simulink model "BiegeMaschineAllein"  (R2015b)
settings: Solver=ode45  StartTime=0.0  StopTime=10  RelTol=1e-3
libraries: simulink x8
settings Model: Creator=taprudho  LastModifiedBy=taprudho
settings DataIOCC: SaveFormat=Array  SignalLoggingSaveFormat=ModelDataLogs
settings OptimizationCC: ExpressionDepthLimit=2147483647
settings DebuggingCC: UnderspecifiedInitializationDetection=Classic  MergeDetectMultiDrivingBlocksExec=none  SolverPrmCheckMsg=warning  FcnCallInpInsideContextMsg=UseLocalSettings  StateNameClashWarn=warning  StrictBusMsg=Warning
settings HardwareCC: ProdBitPerPointer=32  ProdLargestAtomicFloat=None  ProdIntDivRoundTo=Undefined  ProdEndianess=Unspecified  ProdWordSize=32  ProdHWDeviceType=32-bit Generic
settings SFSimCC: SimParseCustomCode=off
settings GRTTargetCC: GeneratePreprocessorConditionals=Disable all  CombineOutputUpdateFcns=off  GRTInterface=on
settings ConfigComp: CovModelRefEnable=Off  CovSFcnEnable=off

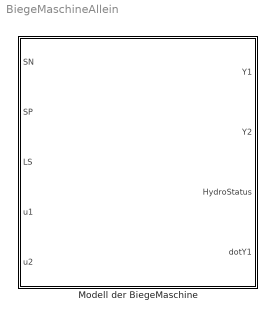
== system BiegeMaschineAllein ==
  Modell der BiegeMaschine : Subsystem

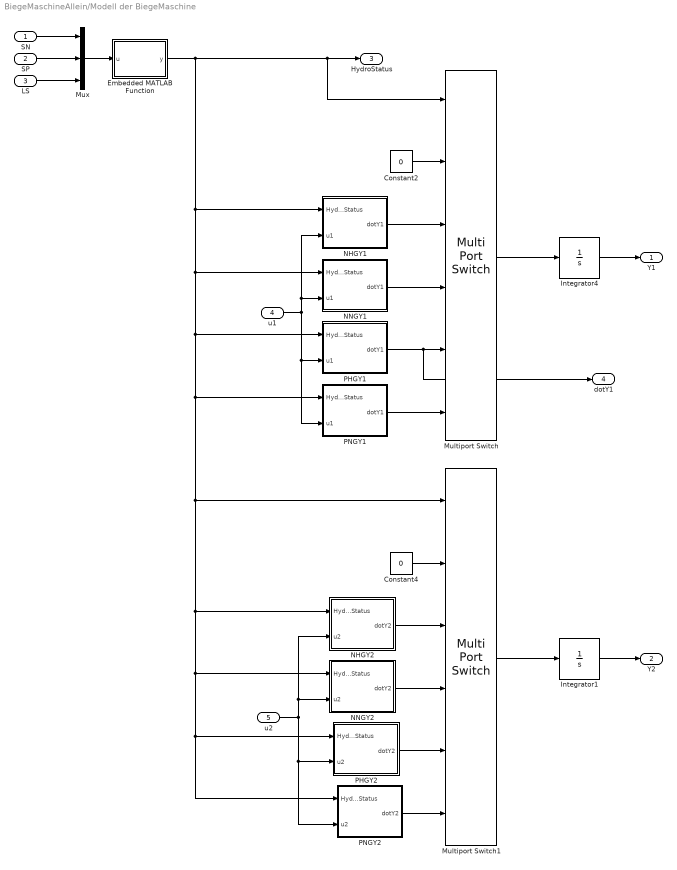
== system BiegeMaschineAllein/Modell der BiegeMaschine ==
  SN : Inport
  SP : Inport  Port=2
  LS : Inport  Port=3
  u1 : Inport  Port=4
  u2 : Inport  Port=5
  Constant2 : Constant  Value=0
  Constant4 : Constant  Value=0
  Embedded MATLAB Function : MATLAB Function  TreatAsAtomicUnit=on
  Integrator1 : Integrator
  Integrator4 : Integrator
  Multiport Switch : MultiPortSwitch  Inputs=5
  Multiport Switch1 : MultiPortSwitch  Inputs=5
  Mux : Mux  Inputs=3
  NHGY1 : Subsystem
  NHGY2 : Subsystem
  NNGY1 : Subsystem
  NNGY2 : Subsystem
  PHGY1 : Subsystem
  PHGY2 : Subsystem
  PNGY1 : Subsystem
  PNGY2 : Subsystem
  Y1 : Outport
  Y2 : Outport  Port=2
  HydroStatus : Outport  Port=3
  dotY1 : Outport  Port=4
  wires:
  SN/1 -> Mux/1
  SP/1 -> Mux/2
  LS/1 -> Mux/3
  Mux/1 -> Embedded MATLAB Function/1(u)
  Embedded MATLAB Function/1(y) -> Multiport Switch/1, HydroStatus/1, NHGY1/1(HydroStatus), NNGY1/1(HydroStatus), PHGY1/1(HydroStatus), Multiport Switch1/1, NHGY2/1(HydroStatus), NNGY2/1(HydroStatus), PHGY2/1(HydroStatus), PNGY2/1(HydroStatus), PNGY1/1(HydroStatus)
  NHGY1/1(dotY1) -> Multiport Switch/3
  NNGY1/1(dotY1) -> Multiport Switch/4
  PHGY1/1(dotY1) -> Multiport Switch/5, dotY1/1
  PNGY1/1(dotY1) -> Multiport Switch/6
  Constant2/1 -> Multiport Switch/2
  Multiport Switch/1 -> Integrator4/1
  Integrator4/1 -> Y1/1
  Constant4/1 -> Multiport Switch1/2
  NHGY2/1(dotY2) -> Multiport Switch1/3
  NNGY2/1(dotY2) -> Multiport Switch1/4
  PHGY2/1(dotY2) -> Multiport Switch1/5
  u2/1 -> NHGY2/2(u2), NNGY2/2(u2), PHGY2/2(u2), PNGY2/2(u2)
  Multiport Switch1/1 -> Integrator1/1
  Integrator1/1 -> Y2/1
  PNGY2/1(dotY2) -> Multiport Switch1/6
  u1/1 -> NHGY1/2(u1), NNGY1/2(u1), PHGY1/2(u1), PNGY1/2(u1)

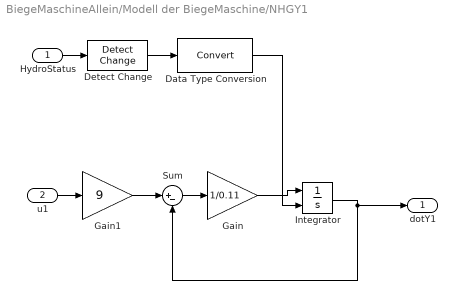
== system BiegeMaschineAllein/Modell der BiegeMaschine/NHGY1 ==
  HydroStatus : Inport
  u1 : Inport  Port=2
  Data Type Conversion : DataTypeConversion
  Detect Change : simulink/Logic and Bit Operations/Detect Change  vinit=0  InputProcessing=Inherited  OutDataTypeStr=uint8
  Gain : Gain  Gain=1/0.11
  Gain1 : Gain  Gain=9
  Integrator : Integrator  ExternalReset=either
  Sum : Sum  Inputs=|+-
  dotY1 : Outport
  wires:
  Gain/1 -> Integrator/1
  Sum/1 -> Gain/1
  Gain1/1 -> Sum/1
  Integrator/1 -> Sum/2, dotY1/1
  HydroStatus/1 -> Detect Change/1
  u1/1 -> Gain1/1
  Detect Change/1 -> Data Type Conversion/1
  Data Type Conversion/1 -> Integrator/2

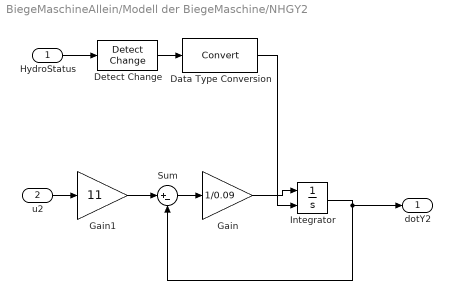
== system BiegeMaschineAllein/Modell der BiegeMaschine/NHGY2 ==
  HydroStatus : Inport
  u2 : Inport  Port=2
  Data Type Conversion : DataTypeConversion
  Detect Change : simulink/Logic and Bit Operations/Detect Change  SystemSampleTime=-1  vinit=0
  Gain : Gain  Gain=1/0.09
  Gain1 : Gain  Gain=11
  Integrator : Integrator  ExternalReset=either
  Sum : Sum  Inputs=|+-
  dotY2 : Outport
  wires:
  Gain/1 -> Integrator/1
  Sum/1 -> Gain/1
  Gain1/1 -> Sum/1
  Integrator/1 -> Sum/2, dotY2/1
  HydroStatus/1 -> Detect Change/1
  u2/1 -> Gain1/1
  Detect Change/1 -> Data Type Conversion/1
  Data Type Conversion/1 -> Integrator/2

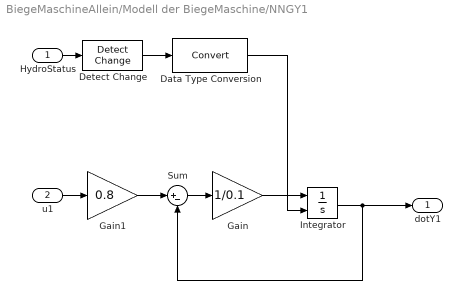
== system BiegeMaschineAllein/Modell der BiegeMaschine/NNGY1 ==
  HydroStatus : Inport
  u1 : Inport  Port=2
  Data Type Conversion : DataTypeConversion
  Detect Change : simulink/Logic and Bit Operations/Detect Change  SystemSampleTime=-1  vinit=0
  Gain : Gain  Gain=1/0.1
  Gain1 : Gain  Gain=0.8
  Integrator : Integrator  ExternalReset=either
  Sum : Sum  Inputs=|+-
  dotY1 : Outport
  wires:
  Gain/1 -> Integrator/1
  Sum/1 -> Gain/1
  Gain1/1 -> Sum/1
  Integrator/1 -> Sum/2, dotY1/1
  Detect Change/1 -> Data Type Conversion/1
  HydroStatus/1 -> Detect Change/1
  u1/1 -> Gain1/1
  Data Type Conversion/1 -> Integrator/2

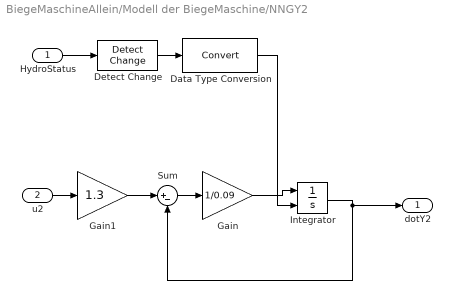
== system BiegeMaschineAllein/Modell der BiegeMaschine/NNGY2 ==
  HydroStatus : Inport
  u2 : Inport  Port=2
  Data Type Conversion : DataTypeConversion
  Detect Change : simulink/Logic and Bit Operations/Detect Change  SystemSampleTime=-1  vinit=0
  Gain : Gain  Gain=1/0.09
  Gain1 : Gain  Gain=1.3
  Integrator : Integrator  ExternalReset=either
  Sum : Sum  Inputs=|+-
  dotY2 : Outport
  wires:
  Gain/1 -> Integrator/1
  Sum/1 -> Gain/1
  Gain1/1 -> Sum/1
  Integrator/1 -> Sum/2, dotY2/1
  HydroStatus/1 -> Detect Change/1
  u2/1 -> Gain1/1
  Detect Change/1 -> Data Type Conversion/1
  Data Type Conversion/1 -> Integrator/2

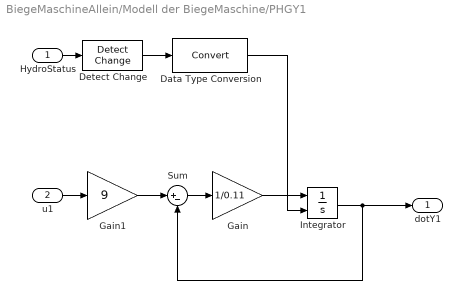
== system BiegeMaschineAllein/Modell der BiegeMaschine/PHGY1 ==
  HydroStatus : Inport
  u1 : Inport  Port=2
  Data Type Conversion : DataTypeConversion
  Detect Change : simulink/Logic and Bit Operations/Detect Change  SystemSampleTime=-1  vinit=0
  Gain : Gain  Gain=1/0.11
  Gain1 : Gain  Gain=9
  Integrator : Integrator  ExternalReset=either
  Sum : Sum  Inputs=|+-
  dotY1 : Outport
  wires:
  Gain/1 -> Integrator/1
  Sum/1 -> Gain/1
  Gain1/1 -> Sum/1
  Integrator/1 -> Sum/2, dotY1/1
  Detect Change/1 -> Data Type Conversion/1
  HydroStatus/1 -> Detect Change/1
  u1/1 -> Gain1/1
  Data Type Conversion/1 -> Integrator/2

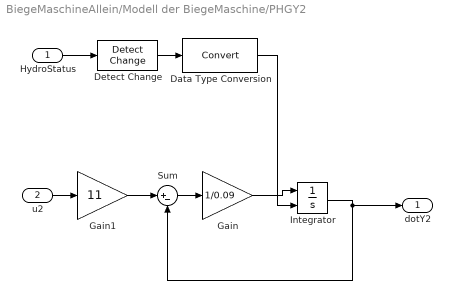
== system BiegeMaschineAllein/Modell der BiegeMaschine/PHGY2 ==
  HydroStatus : Inport
  u2 : Inport  Port=2
  Data Type Conversion : DataTypeConversion
  Detect Change : simulink/Logic and Bit Operations/Detect Change  SystemSampleTime=-1  vinit=0
  Gain : Gain  Gain=1/0.09
  Gain1 : Gain  Gain=11
  Integrator : Integrator  ExternalReset=either
  Sum : Sum  Inputs=|+-
  dotY2 : Outport
  wires:
  Gain/1 -> Integrator/1
  Sum/1 -> Gain/1
  Gain1/1 -> Sum/1
  Integrator/1 -> Sum/2, dotY2/1
  HydroStatus/1 -> Detect Change/1
  u2/1 -> Gain1/1
  Detect Change/1 -> Data Type Conversion/1
  Data Type Conversion/1 -> Integrator/2

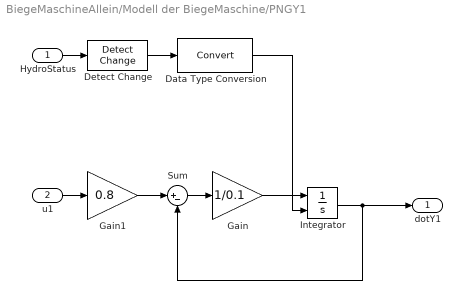
== system BiegeMaschineAllein/Modell der BiegeMaschine/PNGY1 ==
  HydroStatus : Inport
  u1 : Inport  Port=2
  Data Type Conversion : DataTypeConversion
  Detect Change : simulink/Logic and Bit Operations/Detect Change  SystemSampleTime=-1  vinit=0
  Gain : Gain  Gain=1/0.1
  Gain1 : Gain  Gain=0.8
  Integrator : Integrator  ExternalReset=either
  Sum : Sum  Inputs=|+-
  dotY1 : Outport
  wires:
  Gain/1 -> Integrator/1
  Sum/1 -> Gain/1
  Gain1/1 -> Sum/1
  Integrator/1 -> Sum/2, dotY1/1
  u1/1 -> Gain1/1
  Detect Change/1 -> Data Type Conversion/1
  Data Type Conversion/1 -> Integrator/2
  HydroStatus/1 -> Detect Change/1

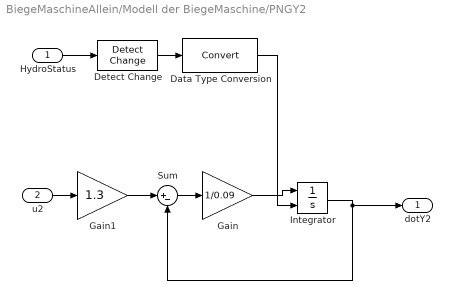
== system BiegeMaschineAllein/Modell der BiegeMaschine/PNGY2 ==
  HydroStatus : Inport
  u2 : Inport  Port=2
  Data Type Conversion : DataTypeConversion
  Detect Change : simulink/Logic and Bit Operations/Detect Change  SystemSampleTime=-1  vinit=0
  Gain : Gain  Gain=1/0.09
  Gain1 : Gain  Gain=1.3
  Integrator : Integrator  ExternalReset=either
  Sum : Sum  Inputs=|+-
  dotY2 : Outport
  wires:
  Gain/1 -> Integrator/1
  Sum/1 -> Gain/1
  Gain1/1 -> Sum/1
  Integrator/1 -> Sum/2, dotY2/1
  HydroStatus/1 -> Detect Change/1
  u2/1 -> Gain1/1
  Detect Change/1 -> Data Type Conversion/1
  Data Type Conversion/1 -> Integrator/2

== matlab function BiegeMaschineAllein/Modell der BiegeMaschine/Embedded MATLAB Function ==
  data: u input; y output
function y  = fcn(u)
% This block supports the Embedded MATLAB subset.
% See the help menu for details. 

% Inputs
SN = u(1);
SP = u(2);
LS = u(3);

% Outputs
STOP = 1;
NHG = 2;
NNG = 3;
PHG = 4;
PNG = 5;


if ((SN > 0.7) && (SP < 0.3) && (LS < 0.3))
    y = NHG;
elseif ((SN > 0.7) && (SP < 0.3) && (LS > 0.7))
    y = NNG;
elseif ((SN < 0.3) && (SP > 0.7) && (LS < 0.3))
    y = PHG;
elseif ((SN < 0.3) && (SP > 0.7) && (LS > 0.7))
    y = PNG;    
else
    y = STOP;
end
